simulink model "body"  (Simulink 7.5)
settings: Solver=ode45  StartTime=0.0  StopTime=10.0  RelTol=1e-3
values from neighbouring files (symbols this model uses):
  del = (Ixx*Izz)-(Ixz*Ixz)    (= 676199)    [valuables.m]
  g = 0.0669    [valuables.m]
  Ixx = 213    [valuables.m]
  Ixz = 88    [valuables.m]
  Iyy = 3310    [valuables.m]
  Izz = 3211    [valuables.m]
undefined symbols (not defined in the file or in its folder): k, m
libraries: vrlib x2
settings Model: Creator=ex08148  LastModifiedBy=ex08148

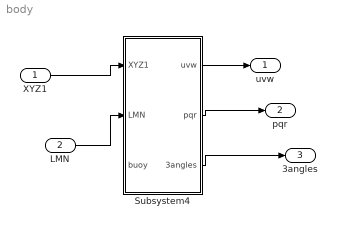
== system body ==
  XYZ1 : Inport
  LMN : Inport  Port=2
  Subsystem4 : Subsystem
  uvw : Outport
  pqr : Outport  Port=2
  3angles : Outport  Port=3
  wires:
  Subsystem4/1(uvw) -> uvw/1
  Subsystem4/2(pqr) -> pqr/1
  XYZ1/1 -> Subsystem4/1(XYZ1)
  LMN/1 -> Subsystem4/2(LMN)
  Subsystem4/3(3angles) -> 3angles/1

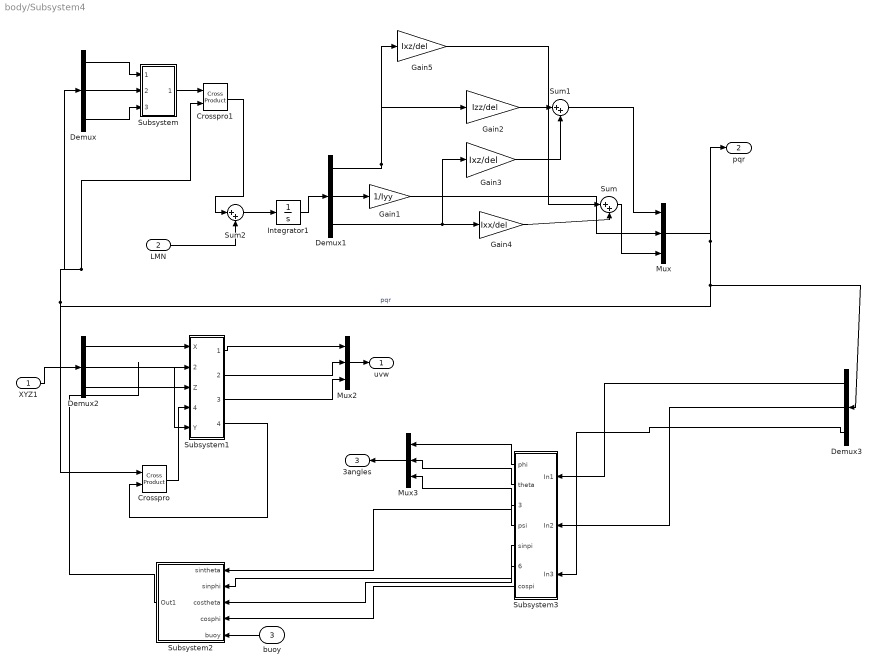
== system body/Subsystem4 ==
  XYZ1 : Inport
  LMN : Inport  Port=2
  buoy : Inport  Port=3
  Crosspro : vrlib/Utilities/Cross Product  SystemSampleTime=-1
  Crosspro1 : vrlib/Utilities/Cross Product  SystemSampleTime=-1
  Demux{,1..3} (4 alike) : Demux  Outputs=3
  Gain1 : Gain  Gain=1/Iyy
  Gain2 : Gain  Gain=Izz/del
  Gain3 : Gain  Gain=Ixz/del
  Gain4 : Gain  Gain=Ixx/del
  Gain5 : Gain  Gain=Ixz/del
  Integrator1 : Integrator
  Mux : Mux  Inputs=3
  Mux2 : Mux  Inputs=3
  Mux3 : Mux  Inputs=3
  Subsystem : Subsystem
  Subsystem1 : Subsystem
  Subsystem2 : Subsystem
  Subsystem3 : Subsystem
  Sum : Sum  Inputs=|++
  Sum1 : Sum  Inputs=|++
  Sum2 : Sum  Inputs=|++
  uvw : Outport
  pqr : Outport  Port=2
  3angles : Outport  Port=3
  wires:
  Mux3/1 -> 3angles/1
  Mux2/1 -> uvw/1
  Demux/2 -> Subsystem/2(In2)
  Demux/1 -> Subsystem/1(In1)
  Demux/3 -> Subsystem/3(In3)
  Demux1/1 -> Gain5/1, Gain2/1
  Demux1/2 -> Gain1/1
  Demux1/3 -> Gain4/1, Gain3/1
  Gain4/1 -> Sum/2
  Gain5/1 -> Sum/1
  Gain2/1 -> Sum1/1
  Gain3/1 -> Sum1/2
  Gain1/1 -> Mux/2
  Sum1/1 -> Mux/1
  Sum/1 -> Mux/3
  Mux/1 -> Demux/1, Crosspro1/2, Crosspro/1, Demux3/1, pqr/1  "pqr"
  Subsystem/1(Out1) -> Crosspro1/1
  Crosspro1/1 -> Sum2/1
  Sum2/1 -> Integrator1/1
  Integrator1/1 -> Demux1/1
  Crosspro/1 -> Subsystem1/4(In5)
  Subsystem1/1(v out) -> Mux2/1
  Subsystem1/2(u out) -> Mux2/2
  Subsystem1/3(w out) -> Mux2/3
  Subsystem1/4(Out4) -> Crosspro/2
  Subsystem2/1(Out1) -> Subsystem1/2(In3)
  Subsystem3/1(phi) -> Mux3/1
  Subsystem3/2(theta) -> Mux3/2
  Demux3/1 -> Subsystem3/1(In1)
  Demux3/2 -> Subsystem3/2(In2)
  Demux3/3 -> Subsystem3/3(In3)
  Subsystem3/3(sinthta) -> Subsystem2/1(sintheta)
  Subsystem3/4(psi) -> Mux3/3
  Subsystem3/6(costhta) -> Subsystem2/3(costheta)
  Subsystem3/7(cospi) -> Subsystem2/4(cosphi)
  Subsystem3/5(sinpi) -> Subsystem2/2(sinphi)
  Demux2/1 -> Subsystem1/1(X)
  Demux2/2 -> Subsystem1/3(Z)
  Demux2/3 -> Subsystem1/5(Y)
  XYZ1/1 -> Demux2/1
  LMN/1 -> Sum2/2
  buoy/1 -> Subsystem2/5(buoy)

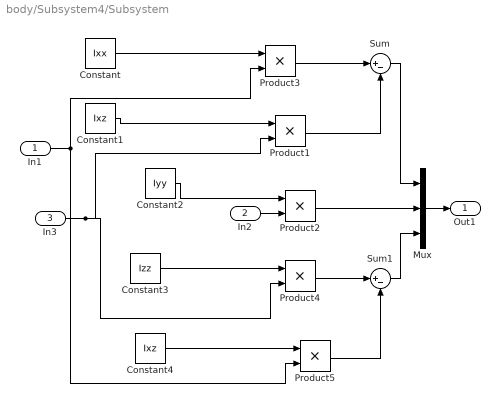
== system body/Subsystem4/Subsystem ==
  In1 : Inport
  In2 : Inport  Port=2
  In3 : Inport  Port=3
  Constant : Constant  Value=Ixx
  Constant1 : Constant  Value=Ixz
  Constant2 : Constant  Value=Iyy
  Constant3 : Constant  Value=Izz
  Constant4 : Constant  Value=Ixz
  Mux : Mux  Inputs=3
  Product{1..5} (5 alike) : Product  RndMeth=Zero
  Sum : Sum  Inputs=|+-
  Sum1 : Sum  Inputs=|+-
  Out1 : Outport
  wires:
  In1/1 -> Product5/2, Product3/2
  Constant4/1 -> Product5/1
  In3/1 -> Product1/2, Product4/2
  Constant3/1 -> Product4/1
  Constant2/1 -> Product2/1
  Constant1/1 -> Product1/1
  Constant/1 -> Product3/1
  Product3/1 -> Sum/1
  Product1/1 -> Sum/2
  Product4/1 -> Sum1/1
  Product5/1 -> Sum1/2
  Product2/1 -> Mux/2
  Sum1/1 -> Mux/3
  Sum/1 -> Mux/1
  Mux/1 -> Out1/1
  In2/1 -> Product2/2

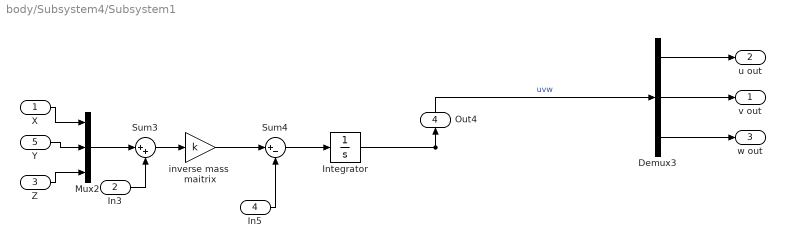
== system body/Subsystem4/Subsystem1 ==
  X : Inport
  In3 : Inport  Port=2
  Z : Inport  Port=3
  In5 : Inport  Port=4
  Y : Inport  Port=5
  Demux3 : Demux  Outputs=3
  Integrator : Integrator
  Mux2 : Mux  Inputs=3
  Sum3 : Sum  Inputs=|++
  Sum4 : Sum  Inputs=|+-
  inverse mass  maitrix : Gain  Gain=k
  v out : Outport
  u out : Outport  Port=2
  w out : Outport  Port=3
  Out4 : Outport  Port=4
  wires:
  Demux3/1 -> u out/1
  Demux3/2 -> v out/1
  Demux3/3 -> w out/1
  Integrator/1 -> Demux3/1, Out4/1  "uvw"
  Sum4/1 -> Integrator/1
  inverse mass  maitrix/1 -> Sum4/1
  Sum3/1 -> inverse mass  maitrix/1
  Mux2/1 -> Sum3/1
  X/1 -> Mux2/1
  In3/1 -> Sum3/2
  Z/1 -> Mux2/3
  In5/1 -> Sum4/2
  Y/1 -> Mux2/2

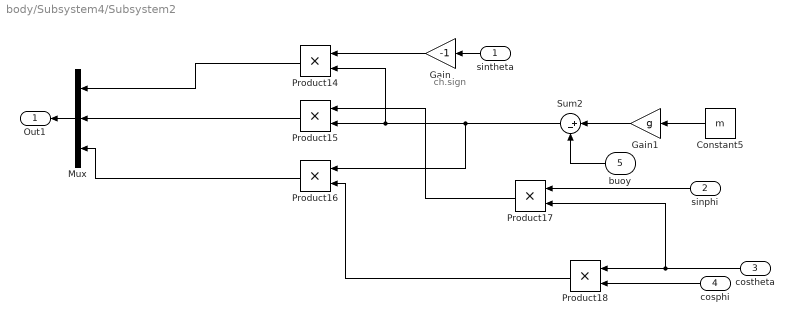
== system body/Subsystem4/Subsystem2 ==
  note: ch.sign
  sintheta : Inport
  sinphi : Inport  Port=2
  costheta : Inport  Port=3
  cosphi : Inport  Port=4
  buoy : Inport  Port=5
  Constant5 : Constant  Value=m
  Gain : Gain  Gain=-1
  Gain1 : Gain  Gain=g
  Mux : Mux  Inputs=3
  Product{14..18} (5 alike) : Product  RndMeth=Zero
  Sum2 : Sum  Inputs=|+-
  Out1 : Outport
  wires:
  Product14/1 -> Mux/1
  Product15/1 -> Mux/2
  Product16/1 -> Mux/3
  Gain/1 -> Product14/1
  Product17/1 -> Product15/1
  Sum2/1 -> Product16/1, Product15/2, Product14/2
  Product18/1 -> Product16/2
  sinphi/1 -> Product17/1
  costheta/1 -> Product18/1, Product17/2
  cosphi/1 -> Product18/2
  sintheta/1 -> Gain/1
  Mux/1 -> Out1/1
  Gain1/1 -> Sum2/1
  Constant5/1 -> Gain1/1
  buoy/1 -> Sum2/2

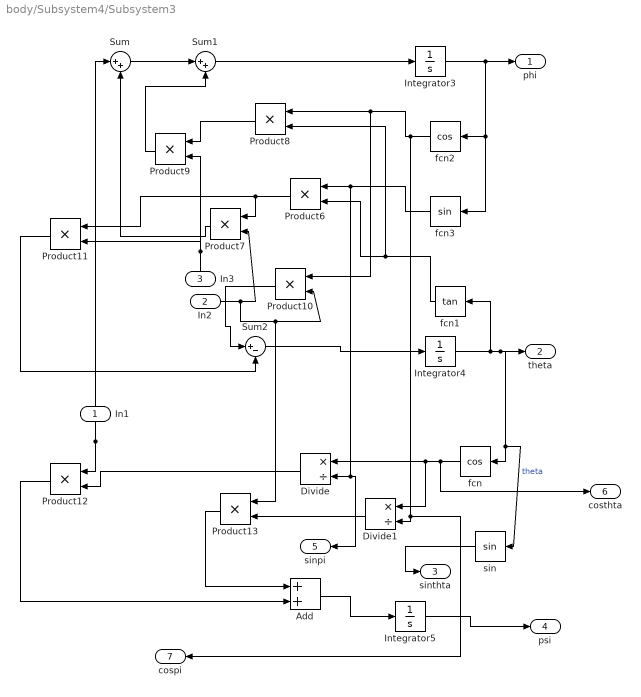
== system body/Subsystem4/Subsystem3 ==
  In1 : Inport
  In2 : Inport  Port=2
  In3 : Inport  Port=3
  Add : Sum  OutDataType=fixdt(1, 16)  OutScaling=2^-10
  Divide : Product  Inputs=*/  OutDataType=fixdt(1, 16)  OutScaling=2^-10
  Divide1 : Product  Inputs=*/  OutDataType=fixdt(1, 16)  OutScaling=2^-10
  Integrator3 : Integrator
  Integrator4 : Integrator
  Integrator5 : Integrator
  Product{6..13} (8 alike) : Product  OutDataType=fixdt(1, 16)  OutScaling=2^0  RndMeth=Zero
  Sum : Sum  Inputs=|++  OutDataType=fixdt(1, 16)  OutScaling=2^0
  Sum1 : Sum  Inputs=|++  OutDataType=fixdt(1, 16)  OutScaling=2^0
  Sum2 : Sum  Inputs=|+-  OutDataType=fixdt(1, 16)  OutScaling=2^0
  fcn : Trigonometry  Operator=cos
  fcn1 : Trigonometry  Operator=tan
  fcn2 : Trigonometry  Operator=cos
  fcn3 : Trigonometry
  sin : Trigonometry
  phi : Outport  OutDataType=fixdt(1, 16)  OutScaling=2^0
  theta : Outport  Port=2  OutDataType=fixdt(1, 16)  OutScaling=2^0
  sinthta : Outport  Port=3  OutDataType=fixdt(1, 16)  OutScaling=2^0
  psi : Outport  Port=4  OutDataType=fixdt(1, 16)  OutScaling=2^0
  sinpi : Outport  Port=5  OutDataType=fixdt(1, 16)  OutScaling=2^0
  costhta : Outport  Port=6  OutDataType=fixdt(1, 16)  OutScaling=2^0
  cospi : Outport  Port=7  OutDataType=fixdt(1, 16)  OutScaling=2^0
  wires:
  Sum/1 -> Sum1/1
  Sum1/1 -> Integrator3/1
  Integrator3/1 -> phi/1, fcn2/1, fcn3/1
  fcn2/1 -> Product8/1, Product10/1, Divide1/2, cospi/1
  fcn3/1 -> Product6/1, Divide/2, sinpi/1
  fcn1/1 -> Product6/2, Product8/2
  Product10/1 -> Sum2/1
  Sum2/1 -> Integrator4/1
  Integrator4/1 -> fcn1/1, theta/1, fcn/1, sin/1  "theta"
  Product8/1 -> Product9/1
  Product9/1 -> Sum1/2
  Product6/1 -> Product11/1, Product7/1
  Product7/1 -> Sum/2
  Product11/1 -> Sum2/2
  fcn/1 -> Divide/1, Divide1/1, costhta/1
  Divide1/1 -> Product13/2
  Product12/1 -> Add/2
  Product13/1 -> Add/1
  In1/1 -> Sum/1, Product12/1
  In2/1 -> Product7/2, Product13/1, Product10/2
  Divide/1 -> Product12/2
  sin/1 -> sinthta/1
  Add/1 -> Integrator5/1
  Integrator5/1 -> psi/1
  In3/1 -> Product11/2, Product9/2
